simulink model "Priklad_4_sim"  (R2022b)
settings: Solver=VariableStepAuto  StartTime=0.0  StopTime=10.0  RelTol=1e-3
settings Model: Creator=honza  LastModifiedBy=honza

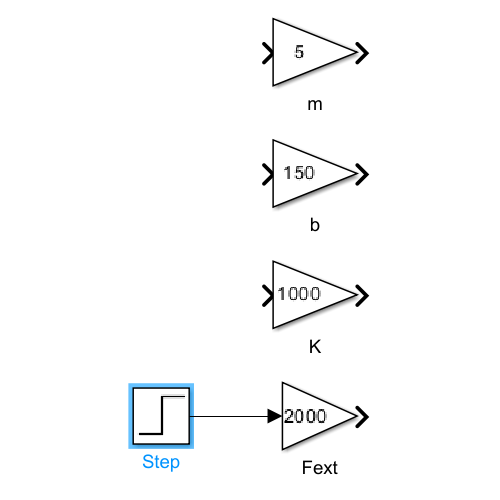
[thumbnail: Simulink's stored preview of the top-level diagram]
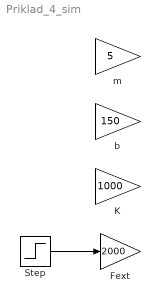
== system Priklad_4_sim ==
  Fext : Gain  Gain=2000
  K : Gain  Gain=1000
  Step : Step  SampleTime=0
  b : Gain  Gain=150
  m : Gain  Gain=5
  wires:
  Step/1 -> Fext/1
